simulink model "EMPlanner_cs2018a"  (R2018a)
settings: Solver=ode5  StartTime=0.0  StopTime=30  FixedStep=1/1000  RelTol=1e-3
PreLoadFcn:
  | mbxruntime.callbacks.PreLoadFcn(bdroot);
PostLoadFcn:
  | mbxruntime.callbacks.PostLoadFcn(bdroot);
InitFcn:
  | mbxruntime.callbacks.InitFcn(bdroot);
StartFcn:
  | mbxruntime.callbacks.StartFcn(bdroot);
StopFcn:
  | mbxruntime.callbacks.StopFcn(bdroot);
model workspace (MAT data in the model file):
  mbox_table : struct (value not decoded)
  model_closed = 0
  sim_status = 0
values from neighbouring files (symbols this model uses):
  aubr = [-8 -7.95 -7.9 -7.85 -7.8 -7.75 -7.7 -7.65 -7.6 -7.55 -7.5 -7.45 ... (261 elements, 1x261)]    [table_calibration.mat]
  tablebr = [-1.5 -1.5 -6.69193204056 -6.72439369683 -6.74529114616 -6.75462438856 -6.75239342402 -6.74076432593 -6.71187451024 -6.7106900587 -6.78609036519 -6.73359919607 ... (261261 elements, 1001x261)]    [table_calibration.mat]
  vubr = [0 0.05 0.1 0.15 0.2 0.25 0.3 0.35 0.4 0.45 0.5 0.55 ... (1001 elements, 1x1001)]    [table_calibration.mat]
undefined symbols (not defined in the file or in its folder): c_factor, cf, cr, DiscIntNeverNeededParam, global_path_x, global_path_y, KD_PID_distance, KD_PID_speed, KI_PID_distance, KI_PID_speed, KP_PID_distance, KP_PID_speed, la, lb, LQR_K1, LQR_K2, LQR_K3, LQR_K4, m, rack_displacement, right_wheel_ground, vx_break_point, warningInitialVelocity, x0
libraries: PreScanSimulinkLibrary x39, simulink x19, simulink_extras x11, Solver_SF x1
(part 4 of 11)

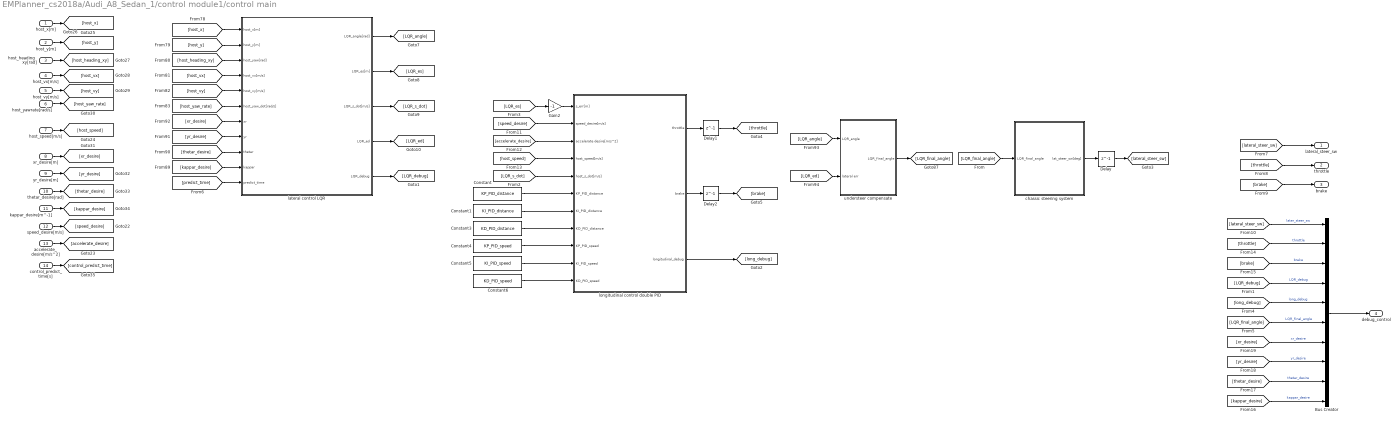
== system EMPlanner_cs2018a/Audi_A8_Sedan_1/control module1/control main ==
  host_x[m] : Inport
  host_y[m] : Inport  Port=2
  host_heading_xy[rad] : Inport  Port=3
  host_vx[m/s] : Inport  Port=4
  host_vy[m/s] : Inport  Port=5
  host_yawrate[rad/s] : Inport  Port=6
  host_speed[m/s] : Inport  Port=7
  xr_desire[m] : Inport  Port=8
  yr_desire[m] : Inport  Port=9
  thetar_desire[rad] : Inport  Port=10
  kappar_desire[m^-1] : Inport  Port=11
  speed_desire[m/s] : Inport  Port=12
  accelerate_desire[m/s^2] : Inport  Port=13
  control_predict_time[s] : Inport  Port=14
  Bus Creator : BusCreator  Inputs=10
  Constant : Constant  Value=KP_PID_distance
  Constant1 : Constant  Value=KI_PID_distance
  Constant3 : Constant  Value=KD_PID_distance
  Constant4 : Constant  Value=KP_PID_speed
  Constant5 : Constant  Value=KI_PID_speed
  Constant6 : Constant  Value=KD_PID_speed
  Delay : Delay  DelayLength=1
  Delay1 : Delay  DelayLength=1
  Delay2 : Delay  DelayLength=1
  Gain2 : Gain  Gain=-1
  chassic steering system : Subsystem
  lateral control LQR : Subsystem
  longitudinal control double PID : Subsystem
  understeer compensate : Subsystem
  lateral_steer_sw : Outport
  throttle : Outport  Port=2
  brake : Outport  Port=3
  debug_control : Outport  Port=4
  wires:
  host_x[m]/1 -> [host_x]
  understeer compensate/1(LQR_final_angle) -> [LQR_final_angle]
  lateral control LQR/1(LQR_angle[rad]) -> [LQR_angle]
  [host_vx] -> lateral control LQR/4(host_vx[m/s])
  thetar_desire[rad]/1 -> [thetar_desire]
  Constant1/1 -> longitudinal control double PID/7(KI_PID_distance)
  [accelerate_desire] -> longitudinal control double PID/3(accelerate desire[m/s^2])
  [host_x] -> lateral control LQR/1(host_x[m])
  [xr_desire] -> lateral control LQR/7(xr)
  accelerate_desire[m/s^2]/1 -> [accelerate_desire]
  [host_y] -> lateral control LQR/2(host_y[m])
  [LQR_s_dot] -> longitudinal control double PID/5(host_s_dot[m/s])
  [yr_desire] -> lateral control LQR/8(yr)
  [LQR_angle] -> understeer compensate/1(LQR_angle)
  xr_desire[m]/1 -> [xr_desire]
  [host_vy] -> lateral control LQR/5(host_vy[m/s])
  lateral control LQR/2(LQR_es[m]) -> [LQR_es]
  host_heading_xy[rad]/1 -> [host_heading_xy]
  [LQR_ed] -> understeer compensate/2(lateral err)
  lateral control LQR/3(LQR_s_dot[m/s]) -> [LQR_s_dot]
  Constant/1 -> longitudinal control double PID/6(KP_PID_distance)
  Constant3/1 -> longitudinal control double PID/8(KD_PID_distance)
  Constant5/1 -> longitudinal control double PID/10(KI_PID_speed)
  Constant4/1 -> longitudinal control double PID/9(KP_PID_speed)
  [host_speed] -> longitudinal control double PID/4(host_speed[m/s])
  [predict_time] -> lateral control LQR/11(predict_time)
  host_vx[m/s]/1 -> [host_vx]
  [speed_desire] -> longitudinal control double PID/2(speed_desire[m/s])
  lateral control LQR/4(LQR_ed) -> [LQR_ed]
  [thetar_desire] -> lateral control LQR/9(thetar)
  [host_heading_xy] -> lateral control LQR/3(host_yaw[rad])
  [kappar_desire] -> lateral control LQR/10(kappar)
  host_yawrate[rad/s]/1 -> [host_yaw_rate]
  kappar_desire[m^-1]/1 -> [kappar_desire]
  yr_desire[m]/1 -> [yr_desire]
  [host_yaw_rate] -> lateral control LQR/6(host_yaw_dot[rad/s])
  host_y[m]/1 -> [host_y]
  host_vy[m/s]/1 -> [host_vy]
  host_speed[m/s]/1 -> [host_speed]
  control_predict_time[s]/1 -> [control_predict_time]
  speed_desire[m/s]/1 -> [speed_desire]
  Constant6/1 -> longitudinal control double PID/11(KD_PID_speed)
  Gain2/1 -> longitudinal control double PID/1(s_err[m])
  [LQR_es] -> Gain2/1
  [LQR_final_angle] -> chassic steering system/1(LQR_final_angle)
  chassic steering system/1(lat_steer_sw[deg]) -> Delay/1
  longitudinal control double PID/1(throttle) -> Delay1/1
  longitudinal control double PID/2(brake) -> Delay2/1
  lateral control LQR/5(LQR_debug) -> [LQR_debug]
  longitudinal control double PID/3(longitudinal_debug) -> [long_debug]
  Delay/1 -> [lateral_steer_sw]
  Delay1/1 -> [throttle]
  Delay2/1 -> [brake]
  [lateral_steer_sw] -> lateral_steer_sw/1
  [throttle] -> throttle/1
  [brake] -> brake/1
  [lateral_steer_sw] -> Bus Creator/1  "later_steer_sw"
  [throttle] -> Bus Creator/2  "throttle"
  [brake] -> Bus Creator/3  "brake"
  [LQR_debug] -> Bus Creator/4  "LQR_debug"
  [long_debug] -> Bus Creator/5  "long_debug"
  [LQR_final_angle] -> Bus Creator/6  "LQR_final_angle"
  Bus Creator/1 -> debug_control/1
  [xr_desire] -> Bus Creator/7  "xr_desire"
  [yr_desire] -> Bus Creator/8  "yr_desire"
  [thetar_desire] -> Bus Creator/9  "thetar_desire"
  [kappar_desire] -> Bus Creator/10  "kappar_desire"

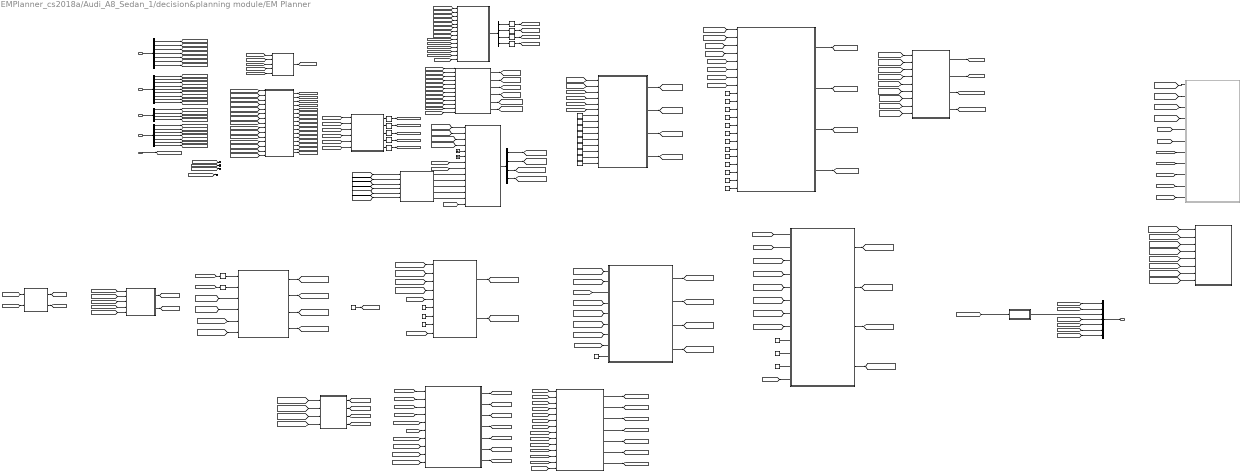
== system EMPlanner_cs2018a/Audi_A8_Sedan_1/decision&planning module/EM Planner ==
  referenceline info : Inport
  location info : Inport  Port=2
  perception info : Inport  Port=3
  pre_planning info : Inport  Port=4
  current time : Inport  Port=5
  Bus Creator : BusCreator  Inputs=7
  Bus Selector : BusSelector  OutputSignals=referenceline_x,referenceline_y,referenceline_heading,referenceline_kappa,origin_match_point_index,origin_x,origin_y
  Bus Selector1 : BusSelector  OutputSignals=host_x,host_y,host_heading_xy,host_vx,host_vy,host_yawrate,host_speed,host_ax,host_ay
  Bus Selector2 : BusSelector  OutputSignals=obs_x_set_gcs,obs_y_set_gcs,obs_velocity_set_gcs,obs_heading_set_gcs
  Bus Selector3 : BusSelector  OutputSignals=trajectory_x_gcs,trajectory_y_gcs,trajectory_heading_gcs,trajectory_kappa_gcs,trajectory_speed_gcs,trajectory_accel_gcs,trajectory_time_gcs
  Bus Selector4 : BusSelector  OutputSignals=s_set,l_set,dl_set,ddl_set
  Bus Selector5 : BusSelector  OutputSignals=s_set,l_set,s_dot_set,l_dot_set
  Cartesian2Frenet : Subsystem
  Cartesian2Frenet1 : Subsystem
  Constant : Constant  Value=1e6
  Constant1 : Constant  Value=2000
  Constant10 : Constant  Value=0.1
  Constant11 : Constant  Value=0.02
  Constant12 : Constant  Value=2
  Constant13 : Constant  Value=25000
  Constant14 : Constant  Value=50
  Constant15 : Constant  Value=20
  Constant{7,16..19,23} (6 alike) : Constant  Value=15
  Constant2 : Constant  Value=2
  Constant20 : Constant  Value=3
  Constant21 : Constant  Value=3
  Constant22 : Constant  Value=1.63
  Constant24 : Constant  Value=4000
  Constant25 : Constant  Value=100
  Constant26 : Constant  Value=10000000
  Constant27 : Constant  Value=0.2*9.8
  Constant28 : Constant  Value=50
  Constant29 : Constant  Value=500
  Constant3 : Constant  Value=3
  Constant4 : Constant  Value=10
  Constant5 : Constant  Value=11
  Constant6 : Constant  Value=4
  Constant8 : Constant
  Constant9 : Constant  Value=10
  Delay : Delay  DelayLength=1
  Delay1 : Delay  DelayLength=1
  Frenet2Cartesian task : MATLAB Function  TreatAsAtomicUnit=on
  Ground : Ground
  Ground1 : Ground
  MATLAB Function : MATLAB Function  TreatAsAtomicUnit=on
  MATLAB Function1 : MATLAB Function  TreatAsAtomicUnit=on
  MATLAB Function2 : MATLAB Function  TreatAsAtomicUnit=on
  MATLAB Function5 : MATLAB Function  TreatAsAtomicUnit=on
  Selector{1..9} (9 alike) : Selector  InputPortWidth=128  IndexOptions=Index vector (dialog)  Indices=1  OutputSizes=1
  Terminator_{1..4} (4 alike) : Terminator
  calc path length and map between point and s : MATLAB Function  TreatAsAtomicUnit=on
  calc plan start info and stitch trajectory : MATLAB Function  TreatAsAtomicUnit=on
  calc speed planning start condition : MATLAB Function  TreatAsAtomicUnit=on
  generate convex space : MATLAB Function  TreatAsAtomicUnit=on
  generate st graph : MATLAB Function  TreatAsAtomicUnit=on
  genrate index to s : MATLAB Function  TreatAsAtomicUnit=on
  increase st point count : MATLAB Function  TreatAsAtomicUnit=on
  obs : Subsystem
  path and speed merge : MATLAB Function  TreatAsAtomicUnit=on
  path decision task : Subsystem
  path planning task : Subsystem
  plot : MATLAB Function  Commented=on  TreatAsAtomicUnit=on
  spee planning with quadratic programming (qp) : MATLAB Function  TreatAsAtomicUnit=on
  speed decision with dynamic planning(dp) : MATLAB Function  TreatAsAtomicUnit=on
  stitch trajectory : MATLAB Function  TreatAsAtomicUnit=on
  EM Planner result : Outport
  wires:
  referenceline info/1 -> Bus Selector/1
  location info/1 -> Bus Selector1/1
  perception info/1 -> Bus Selector2/1
  pre_planning info/1 -> Bus Selector3/1
  current time/1 -> [current_time]
  Bus Selector3/1 -> [pre_trajectory_x_gcs]  "<trajectory_x_gcs>"
  Bus Selector3/2 -> [pre_trajectory_y_gcs]  "<trajectory_y_gcs>"
  Bus Selector3/3 -> [pre_trajectory_heading_gcs]  "<trajectory_heading_gcs>"
  Bus Selector3/4 -> [pre_trajectory_kappa_gcs]  "<trajectory_kappa_gcs>"
  Bus Selector3/5 -> [pre_trajectory_speed_gcs]  "<trajectory_speed_gcs>"
  Bus Selector3/6 -> [pre_trajectory_accel_gcs]  "<trajectory_accel_gcs>"
  Bus Selector3/7 -> [pre_trajectory_time]  "<trajectory_time_gcs>"
  Bus Selector2/1 -> [obs_x_set_gcs]  "<obs_x_set_gcs>"
  Bus Selector2/2 -> [obs_y_set_gcs]  "<obs_y_set_gcs>"
  Bus Selector2/3 -> [obs_velocity_set_gcs]  "<obs_velocity_set_gcs>"
  Bus Selector2/4 -> [obs_heading_set_gcs]  "<obs_heading_set_gcs>"
  Bus Selector1/1 -> [host_x]  "<host_x>"
  Bus Selector1/2 -> [host_y]  "<host_y>"
  Bus Selector1/3 -> [host_heading_xy]  "<host_heading_xy>"
  Bus Selector1/4 -> [host_vx_vcs]  "<host_vx>"
  Bus Selector1/5 -> [host_vy_vcs]  "<host_vy>"
  Bus Selector1/6 -> [host_yawrate]  "<host_yawrate>"
  Bus Selector1/7 -> [host_speed]  "<host_speed>"
  Bus Selector1/8 -> [host_ax_vcs]  "<host_ax>"
  Bus Selector1/9 -> [host_ay_vcs]  "<host_ay>"
  Bus Selector/1 -> [referenceline_x]  "<referenceline_x>"
  Bus Selector/2 -> [referenceline_y]  "<referenceline_y>"
  Bus Selector/3 -> [referenceline_heading]  "<referenceline_heading>"
  Bus Selector/4 -> [referenceline_kappa]  "<referenceline_kappa>"
  [host_ay_vcs] -> calc plan start info and stitch trajectory/15(host_ay)
  [host_ax_vcs] -> calc plan start info and stitch trajectory/14(host_ax)
  [host_vy_vcs] -> calc plan start info and stitch trajectory/13(host_vy)
  [host_vx_vcs] -> calc plan start info and stitch trajectory/12(host_vx)
  [host_heading_xy] -> calc plan start info and stitch trajectory/11(host_heading_xy)
  [host_y] -> calc plan start info and stitch trajectory/10(host_y)
  [host_x] -> calc plan start info and stitch trajectory/9(host_x)
  [current_time] -> calc plan start info and stitch trajectory/8(current_time)
  [pre_trajectory_x_gcs] -> calc plan start info and stitch trajectory/1(pre_trajectory_x)
  [pre_trajectory_y_gcs] -> calc plan start info and stitch trajectory/2(pre_trajectory_y)
  [pre_trajectory_time] -> calc plan start info and stitch trajectory/7(pre_trajectory_time)
  [pre_trajectory_accel_gcs] -> calc plan start info and stitch trajectory/6(pre_trajectory_accel)
  [pre_trajectory_speed_gcs] -> calc plan start info and stitch trajectory/5(pre_trajectory_velocity)
  [pre_trajectory_kappa_gcs] -> calc plan start info and stitch trajectory/4(pre_trajectory_kappa)
  [pre_trajectory_heading_gcs] -> calc plan start info and stitch trajectory/3(pre_trajectory_heading)
  calc plan start info and stitch trajectory/1(plan_start_x) -> [plan_start_x_gcs]
  calc plan start info and stitch trajectory/2(plan_start_y) -> [plan_start_y_gcs]
  calc plan start info and stitch trajectory/3(plan_start_heading) -> [plan_start_heading_gcs]
  calc plan start info and stitch trajectory/4(plan_start_kappa) -> [plan_start_kappa_gcs]
  calc plan start info and stitch trajectory/5(plan_start_vx) -> [plan_start_vx_gcs]
  calc plan start info and stitch trajectory/6(plan_start_vy) -> [plan_start_vy_gcs]
  calc plan start info and stitch trajectory/7(plan_start_ax) -> [plan_start_ax_gcs]
  calc plan start info and stitch trajectory/8(plan_start_ay) -> [plan_start_ay_gcs]
  calc plan start info and stitch trajectory/9(plan_start_time) -> [plan_start_time]
  calc plan start info and stitch trajectory/10(stitch_x) -> [stitch_x_gcs]
  calc plan start info and stitch trajectory/11(stitch_y) -> [stitch_y_gcs]
  calc plan start info and stitch trajectory/12(stitch_heading) -> [stitch_heading_gcs]
  calc plan start info and stitch trajectory/13(stitch_kappa) -> [stitch_kappa_gcs]
  calc plan start info and stitch trajectory/14(stitch_speed) -> [stitch_speed_gcs]
  calc plan start info and stitch trajectory/15(stitch_accel) -> [stitch_accel_gcs]
  calc plan start info and stitch trajectory/16(stitch_time) -> [stitch_time]
  Bus Selector/5 -> [origin_match_point_index]  "<origin_match_point_index>"
  Bus Selector/6 -> [origin_x]  "<origin_x>"
  Bus Selector/7 -> [origin_y]  "<origin_y>"
  [referenceline_x] -> genrate index to s/1(path_x)
  [referenceline_y] -> genrate index to s/2(path_y)
  [origin_x] -> genrate index to s/3(origin_x)
  [origin_y] -> genrate index to s/4(origin_y)
  [origin_match_point_index] -> genrate index to s/5(origin_match_point_index)
  genrate index to s/1(index2s) -> [index2s]
  MATLAB Function2/5(proj_kappa_set) -> Selector5/1
  MATLAB Function2/3(proj_y_set) -> Selector3/1
  MATLAB Function2/1(match_point_index_set) -> Selector1/1
  MATLAB Function2/4(proj_heading_set) -> Selector4/1
  MATLAB Function2/2(proj_x_set) -> Selector2/1
  [plan_start_x_gcs] -> MATLAB Function2/1(x_set)
  [plan_start_y_gcs] -> MATLAB Function2/2(y_set)
  [referenceline_x] -> MATLAB Function2/3(frenet_path_x)
  [referenceline_y] -> MATLAB Function2/4(frenet_path_y)
  [referenceline_heading] -> MATLAB Function2/5(frenet_path_heading)
  [referenceline_kappa] -> MATLAB Function2/6(frenet_path_kappa)
  Selector1/1 -> [plan_start_match_point_index]
  Selector2/1 -> [plan_start_proj_x]
  Selector3/1 -> [plan_start_proj_y]
  Selector4/1 -> [plan_start_proj_heading]
  Selector5/1 -> [plan_start_proj_kappa]
  [plan_start_y_gcs] -> Cartesian2Frenet/2(y_set)
  [plan_start_x_gcs] -> Cartesian2Frenet/1(x_set)
  [plan_start_vx_gcs] -> Cartesian2Frenet/3(vx_set)
  [plan_start_vy_gcs] -> Cartesian2Frenet/4(vy_set)
  [plan_start_ax_gcs] -> Cartesian2Frenet/5(ax_set)
  [plan_start_ay_gcs] -> Cartesian2Frenet/6(ay_set)
  [referenceline_x] -> Cartesian2Frenet/7(frenet_path_x)
  [referenceline_y] -> Cartesian2Frenet/8(frenet_path_y)
  [plan_start_match_point_index] -> Cartesian2Frenet/9(proj_match_point_index_set)
  [plan_start_proj_x] -> Cartesian2Frenet/10(proj_x_set)
  [plan_start_proj_y] -> Cartesian2Frenet/11(proj_y_set)
  [plan_start_proj_heading] -> Cartesian2Frenet/12(proj_heading_set)
  [plan_start_proj_kappa] -> Cartesian2Frenet/13(proj_kappa_set)
  Cartesian2Frenet/1(Cartesian2FrenetOut) -> Bus Selector4/1
  Bus Selector4/4 -> Selector9/1  "<ddl_set>"
  Bus Selector4/3 -> Selector8/1  "<dl_set>"
  Bus Selector4/2 -> Selector7/1  "<l_set>"
  Bus Selector4/1 -> Selector6/1  "<s_set>"
  Selector6/1 -> [plan_start_s]
  Selector7/1 -> [plan_start_l]
  Selector8/1 -> [plan_start_dl]
  Selector9/1 -> [plan_start_ddl]
  [index2s] -> Cartesian2Frenet/14(index2s)
  [host_x] -> obs/1(host_x)
  [host_y] -> obs/2(host_y)
  [host_heading_xy] -> obs/3(host_heading_xy)
  [obs_x_set_gcs] -> obs/4(obs_x_set_gcs)
  [obs_y_set_gcs] -> obs/5(obs_y_set_gcs)
  [obs_velocity_set_gcs] -> obs/6(obs_velocity_set_gcs)
  [obs_heading_set_gcs] -> obs/7(obs_heading_set_gcs)
  [referenceline_x] -> obs/8(referenceline_x)
  [referenceline_y] -> obs/9(referenceline_y)
  [referenceline_heading] -> obs/10(referenceline_heading)
  [referenceline_kappa] -> obs/11(referenceline_kappa)
  [index2s] -> obs/12(index2s)
  obs/1(static_obs_s_set) -> [static_obs_s_set]
  obs/2(static_obs_l_set) -> [static_obs_l_set]
  path and speed merge/7(trajectory_time) -> [trajectory_time]
  path and speed merge/1(trajectory_x) -> [trajectory_x]
  [trajectory_speed] -> stitch trajectory/5(trajectory_speed)
  path and speed merge/4(trajectory_kappa) -> [trajectory_kappa]
  [plan_start_vy_gcs] -> calc speed planning start condition/2(plan_start_vy)
  [stitch_time] -> stitch trajectory/14(stitch_time)
  calc path length and map between point and s/2(path_index2s) -> [path_index2s]
  [plan_start_heading_gcs] -> calc speed planning start condition/5(plan_start_heading)
  Bus Creator/1 -> EM Planner result/1
  [trajectory_x_final] -> Bus Creator/1  "trajectory_x_gcs"
  stitch trajectory/4(trajectory_kappa_final) -> [trajectory_kappa_final]
  [plan_start_ax_gcs] -> calc speed planning start condition/3(plan_start_ax)
  calc speed planning start condition/1(plan_start_s_dot) -> [plan_start_s_dot]
  [plan_start_ay_gcs] -> calc speed planning start condition/4(plan_start_ay)
  [stitch_speed_gcs] -> stitch trajectory/12(stitch_speed)
  [trajectory_time_final] -> Bus Creator/7  "trajectory_time_gcs"
  [stitch_x_gcs] -> stitch trajectory/8(stitch_x)
  stitch trajectory/1(trajectory_x_final) -> [trajectory_x_final]
  [trajectory_accel_final] -> Bus Creator/6  "trajectory_accel_gcs"
  [stitch_heading_gcs] -> stitch trajectory/10(stitch_heading)
  [trajectory_speed_final] -> Bus Creator/5  "trajectory_speed_gcs"
  [stitch_y_gcs] -> stitch trajectory/9(stitch_y)
  stitch trajectory/6(trajectory_accel_final) -> [trajectory_accel_final]
  [plan_start_vx_gcs] -> calc speed planning start condition/1(plan_start_vx)
  [trajectory_heading_final] -> MATLAB Function/1(trajectory_heading_final)
  [trajectory_accel] -> stitch trajectory/6(trajectory_accel)
  [trajectory_kappa] -> stitch trajectory/4(trajectory_kappa)
  [trajectory_x_init] -> path and speed merge/7(trajectory_x_init)
  stitch trajectory/2(trajectory_y_final) -> [trajectory_y_final]
  stitch trajectory/3(trajectory_heading_final) -> [trajectory_heading_final]
  [trajectory_kappa_final] -> Bus Creator/4  "trajectory_kappa_gcs"
  path and speed merge/3(trajectory_heading) -> [trajectory_heading]
  stitch trajectory/5(trajectory_speed_final) -> [trajectory_speed_final]
  [trajectory_y_final] -> Bus Creator/2  "trajectory_y_gcs"
  [trajectory_y] -> stitch trajectory/2(trajectory_y)
  calc path length and map between point and s/1(path_s_end) -> [path_s_end]
  calc speed planning start condition/2(plan_start_s_dot2) -> [plan_start_s_dot2]
  [trajectory_kappa_init] -> path and speed merge/10(trajectory_kappa_init)
  [stitch_accel_gcs] -> stitch trajectory/13(stitch_accel)
  [trajectory_x] -> stitch trajectory/1(trajectory_x)
  [trajectory_y_init] -> calc path length and map between point and s/2(trajectory_y)
  path and speed merge/6(trajectory_accel) -> [trajectory_accel]
  [stitch_kappa_gcs] -> stitch trajectory/11(stitch_kappa)
  [path_index2s] -> path and speed merge/6(path_s)
  path and speed merge/2(trajectory_y) -> [trajectory_y]
  [trajectory_heading_init] -> path and speed merge/9(trajectory_heading_init)
  [plan_start_time] -> path and speed merge/5(current_time)
  path and speed merge/5(trajectory_speed) -> [trajectory_speed]
  [trajectory_y_init] -> path and speed merge/8(trajectory_y_init)
  [trajectory_time] -> stitch trajectory/7(trajectory_time)
  [trajectory_heading] -> stitch trajectory/3(trajectory_heading)
  [trajectory_x_init] -> calc path length and map between point and s/1(trajectory_x)
  [index2s] -> Frenet2Cartesian task/9(index2s)
  [referenceline_x] -> Frenet2Cartesian task/5(frenet_path_x)
  [referenceline_y] -> Frenet2Cartesian task/6(frenet_path_y)
  [referenceline_heading] -> Frenet2Cartesian task/7(frenet_path_heading)
  [referenceline_kappa] -> Frenet2Cartesian task/8(frenet_path_kappa)
  Frenet2Cartesian task/1(x_set) -> [trajectory_x_init]
  Frenet2Cartesian task/2(y_set) -> [trajectory_y_init]
  Frenet2Cartesian task/3(heading_set) -> [trajectory_heading_init]
  Frenet2Cartesian task/4(kappa_set) -> [trajectory_kappa_init]
  [dp_path_s_final] -> plot/1(dp_s)
  [dp_path_l_final] -> plot/2(dp_l)
  [l_min] -> plot/5(l_min)
  [l_max] -> plot/6(l_max)
  [plan_start_dl] -> plot/11(start_dl)
  [plan_start_l] -> plot/10(start_l)
  [plan_start_s] -> plot/9(start_s)
  [static_obs_s_set] -> plot/7(obs_s_set)
  [static_obs_l_set] -> plot/8(obs_l_set)
  path decision task/1(dp_path_s_final) -> [dp_path_s_final]
  path decision task/2(dp_path_l_final) -> [dp_path_l_final]
  path decision task/3(dp_path_dl_final) -> [dp_path_dl_final]
  path decision task/4(dp_path_ddl_final) -> [dp_path_ddl_final]
  [static_obs_s_set] -> path decision task/1(static_obs_s_set)
  [static_obs_l_set] -> path decision task/2(static_obs_l_set)
  [plan_start_ddl] -> path decision task/6(plan_start_ddl)
  [plan_start_dl] -> path decision task/5(plan_start_dl)
  [plan_start_l] -> path decision task/4(plan_start_l)
  [plan_start_s] -> path decision task/3(plan_start_s)
  [dp_path_s_final] -> path planning task/1(dp_path_s_final)
  [dp_path_l_final] -> path planning task/2(dp_path_l_final)
  [plan_start_l] -> path planning task/6(plan_start_l)
  [plan_start_ddl] -> path planning task/8(plan_start_ddl)
  [plan_start_dl] -> path planning task/7(plan_start_dl)
  Constant22/1 -> path planning task/19(host_w)
  Constant21/1 -> path planning task/18(host_d2)
  Constant20/1 -> path planning task/17(host_d1)
  Constant19/1 -> path planning task/16(qp_cost_end_ddl)
  Constant18/1 -> path planning task/15(qp_cost_end_dl)
  Constant17/1 -> path planning task/14(qp_cost_endl)
  Constant16/1 -> path planning task/13(qp_cost_centre)
  Constant15/1 -> path planning task/12(qp_cost_dddl)
  Constant14/1 -> path planning task/11(qp_cost_ddl)
  Constant13/1 -> path planning task/10(qp_cost_dl)
  Constant12/1 -> path planning task/9(qp_cost_l)
  Constant8/1 -> path decision task/15(dp_sample_l)
  Constant7/1 -> path decision task/14(dp_sample_s)
  Constant6/1 -> path decision task/13(dp_col)
  Constant5/1 -> path decision task/12(dp_row)
  Constant4/1 -> path decision task/11(dp_cost_ref)
  Constant3/1 -> path decision task/10(dp_cost_dddl)
  Constant/1 -> path decision task/7(dp_cost_collision)
  Constant1/1 -> path decision task/8(dp_cost_dl)
  Constant2/1 -> path decision task/9(dp_cost_ddl)
  [static_obs_s_set] -> path planning task/3(static_obs_s_set)
  [static_obs_l_set] -> path planning task/4(static_obs_l_set)
  Constant10/1 -> path planning task/20(delta_dl_max)
  Constant11/1 -> path planning task/21(delta_ddl_max)
  path planning task/1(qp_path_s_final) -> [qp_path_s_final]
  path planning task/2(qp_path_l_final) -> [qp_path_l_final]
  path planning task/3(qp_path_dl_final) -> [qp_path_dl_final]
  path planning task/4(qp_path_ddl_final) -> [qp_path_ddl_final]
  [qp_path_ddl_final] -> Frenet2Cartesian task/4(ddl_set)
  [qp_path_l_final] -> Frenet2Cartesian task/2(l_set)
  [qp_path_dl_final] -> Frenet2Cartesian task/3(dl_set)
  [qp_path_s_final] -> Frenet2Cartesian task/1(s_set)
  [qp_path_s_final] -> plot/3(qp_s)
  [qp_path_l_final] -> plot/4(qp_l)
  [plan_start_s] -> path planning task/5(plan_start_s)
  MATLAB Function/1(y) -> Bus Creator/3  "trajectory_heading_gcs"
  obs/3(dynamic_obs_x_set) -> [dynamic_obs_x_set]
  obs/4(dynamic_obs_y_set) -> [dynamic_obs_y_set]
  obs/5(dynamic_obs_vx_set) -> [dynamic_obs_vx_set]
  obs/6(dynamic_obs_vy_set) -> [dynamic_obs_vy_set]
  increase st point count/3(s_dot2) -> [s_dot2]
  increase st point count/2(s_dot) -> [s_dot]
  increase st point count/1(s) -> [s]
  increase st point count/4(relative_time) -> [relative_time]
  [s_dot] -> path and speed merge/2(s_dot)
  [s] -> path and speed merge/1(s)
  [s_dot2] -> path and speed merge/3(s_dot2)
  [relative_time] -> path and speed merge/4(relative_time)
  [dynamic_obs_vy_set] -> Cartesian2Frenet1/4(vy_set)
  [dynamic_obs_vx_set] -> Cartesian2Frenet1/3(vx_set)
  [dynamic_obs_y_set] -> Cartesian2Frenet1/2(y_set)
  [dynamic_obs_x_set] -> Cartesian2Frenet1/1(x_set)
  Ground/1 -> Cartesian2Frenet1/5(ax_set)
  Ground1/1 -> Cartesian2Frenet1/6(ay_set)
  [trajectory_x_init] -> Cartesian2Frenet1/7(frenet_path_x)
  [trajectory_y_init] -> Cartesian2Frenet1/8(frenet_path_y)
  MATLAB Function1/1(match_point_index_set) -> Cartesian2Frenet1/9(proj_match_point_index_set)
  MATLAB Function1/2(proj_x_set) -> Cartesian2Frenet1/10(proj_x_set)
  MATLAB Function1/3(proj_y_set) -> Cartesian2Frenet1/11(proj_y_set)
  MATLAB Function1/4(proj_heading_set) -> Cartesian2Frenet1/12(proj_heading_set)
  MATLAB Function1/5(proj_kappa_set) -> Cartesian2Frenet1/13(proj_kappa_set)
  [trajectory_x_init] -> MATLAB Function1/3(frenet_path_x)
  [trajectory_y_init] -> MATLAB Function1/4(frenet_path_y)
  [trajectory_heading_init] -> MATLAB Function1/5(frenet_path_heading)
  [trajectory_kappa_init] -> MATLAB Function1/6(frenet_path_kappa)
  [dynamic_obs_y_set] -> MATLAB Function1/2(y_set)
  [dynamic_obs_x_set] -> MATLAB Function1/1(x_set)
  Cartesian2Frenet1/1(Cartesian2FrenetOut) -> Bus Selector5/1
  Bus Selector5/1 -> [dynamic_obs_s_set]  "<s_set>"
  Bus Selector5/2 -> [dynamic_obs_l_set]  "<l_set>"
  Bus Selector5/3 -> [dynamic_obs_s_dot_set]  "<s_dot_set>"
  Bus Selector5/4 -> [dynamic_obs_l_dot_set]  "<l_dot_set>"
  [path_index2s] -> Cartesian2Frenet1/14(index2s)
  [s] -> Delay/1
  [relative_time] -> Delay1/1
  Delay/1 -> generate st graph/1(pre_trajectory_s)
  Delay1/1 -> generate st graph/2(pre_trajectory_t)
  stitch trajectory/7(trajectory_time_final) -> [trajectory_time_final]
  [dynamic_obs_s_set] -> generate st graph/3(dynamic_obs_s_set)
  [dynamic_obs_l_set] -> generate st graph/4(dynamic_obs_l_set)
  [dynamic_obs_s_dot_set] -> generate st graph/5(dynamic_obs_s_dot_set)
  [dynamic_obs_l_dot_set] -> generate st graph/6(dynamic_obs_l_dot_set)
  generate st graph/1(obs_st_s_in_set) -> [obs_st_s_in_set]
  generate st graph/3(obs_st_t_in_set) -> [obs_st_t_in_set]
  generate st graph/4(obs_st_t_out_set) -> [obs_st_t_out_set]
  generate st graph/2(obs_st_s_out_set) -> [obs_st_s_out_set]
  [obs_st_s_in_set] -> speed decision with dynamic planning(dp)/1(obs_st_s_in_set)
  [obs_st_s_out_set] -> speed decision with dynamic planning(dp)/2(obs_st_s_out_set)
  [obs_st_t_in_set] -> speed decision with dynamic planning(dp)/3(obs_st_t_in_set)
  [obs_st_t_out_set] -> speed decision with dynamic planning(dp)/4(obs_st_t_out_set)
  Constant24/1 -> speed decision with dynamic planning(dp)/6(w_cost_ref_speed)
  Constant25/1 -> speed decision with dynamic planning(dp)/7(w_cost_accel)
  Constant26/1 -> speed decision with dynamic planning(dp)/8(w_cost_obs)
  [plan_start_s_dot] -> speed decision with dynamic planning(dp)/9(plan_start_s_dot)
  [path_index2s] -> generate convex space/3(path_index2s)
  speed decision with dynamic planning(dp)/2(dp_speed_t) -> [dp_speed_t]
  [dp_speed_s] -> generate convex space/1(dp_speed_s)
  [dp_speed_t] -> generate convex space/2(dp_speed_t)
  [obs_st_s_in_set] -> generate convex space/4(obs_st_s_in_set)
  [obs_st_t_out_set] -> generate convex space/7(obs_st_t_out_set)
  [obs_st_t_in_set] -> generate convex space/6(obs_st_t_in_set)
  [obs_st_s_out_set] -> generate convex space/5(obs_st_s_out_set)
  [trajectory_kappa_init] -> generate convex space/8(trajectory_kappa_init)
  Constant27/1 -> generate convex space/9(max_lateral_accel)
  generate convex space/1(s_lb) -> [s_lb]
  generate convex space/2(s_ub) -> [s_ub]
  generate convex space/3(s_dot_lb) -> [s_dot_lb]
  generate convex space/4(s_dot_ub) -> [s_dot_ub]
  speed decision with dynamic planning(dp)/1(dp_speed_s) -> [dp_speed_s]
  [obs_st_s_in_set] -> MATLAB Function5/5(obs_s_in_set)
  [obs_st_s_out_set] -> MATLAB Function5/6(obs_s_out_set)
  [obs_st_t_in_set] -> MATLAB Function5/7(obs_t_in_set)
  [obs_st_t_out_set] -> MATLAB Function5/8(obs_t_out_set)
  [plan_start_s_dot] -> spee planning with quadratic programming (qp)/1(plan_start_s_dot)
  [dp_speed_s] -> spee planning with quadratic programming (qp)/3(dp_speed_s)
  [dp_speed_t] -> spee planning with quadratic programming (qp)/4(dp_speed_t)
  [s_lb] -> spee planning with quadratic programming (qp)/5(s_lb)
  [s_ub] -> spee planning with quadratic programming (qp)/6(s_ub)
  [s_dot_lb] -> spee planning with quadratic programming (qp)/7(s_dot_lb)
  [s_dot_ub] -> spee planning with quadratic programming (qp)/8(s_dot_ub)
  spee planning with quadratic programming (qp)/1(qp_s_init) -> [qp_s_init]
  spee planning with quadratic programming (qp)/2(qp_s_dot_init) -> [qp_s_dot_init]
  spee planning with quadratic programming (qp)/3(qp_s_dot2_init) -> [qp_s_dot2_init]
  spee planning with quadratic programming (qp)/4(relative_time_init) -> [relative_time_init]
  [qp_s_init] -> increase st point count/1(s_init)
  [qp_s_dot2_init] -> increase st point count/3(s_dot2_init)
  [qp_s_dot_init] -> increase st point count/2(s_dot_init)
  [relative_time_init] -> increase st point count/4(relative_time_init)
  Constant9/1 -> spee planning with quadratic programming (qp)/9(w_cost_s_dot2)
  Constant28/1 -> spee planning with quadratic programming (qp)/10(w_cost_v_ref)
  Constant29/1 -> spee planning with quadratic programming (qp)/11(w_cost_jerk)
  [plan_start_s_dot2] -> spee planning with quadratic programming (qp)/2(plan_start_s_dot2)
  [dp_speed_t] -> MATLAB Function5/2(dp_speed_t)
  [dp_speed_s] -> MATLAB Function5/1(dp_speed_s)
  [qp_s_init] -> MATLAB Function5/3(qp_speed_s)
  [relative_time_init] -> MATLAB Function5/4(qp_speed_t)
  Constant23/1 -> [reference_speed]
  [reference_speed] -> speed decision with dynamic planning(dp)/5(reference_speed_unlimit)
  [reference_speed] -> spee planning with quadratic programming (qp)/12(speed_reference)
  [pre_trajectory_x_gcs] -> Terminator_1/1
  [pre_trajectory_y_gcs] -> Terminator_2/1
  [pre_trajectory_speed_gcs] -> Terminator_3/1
  [pre_trajectory_time] -> Terminator_4/1

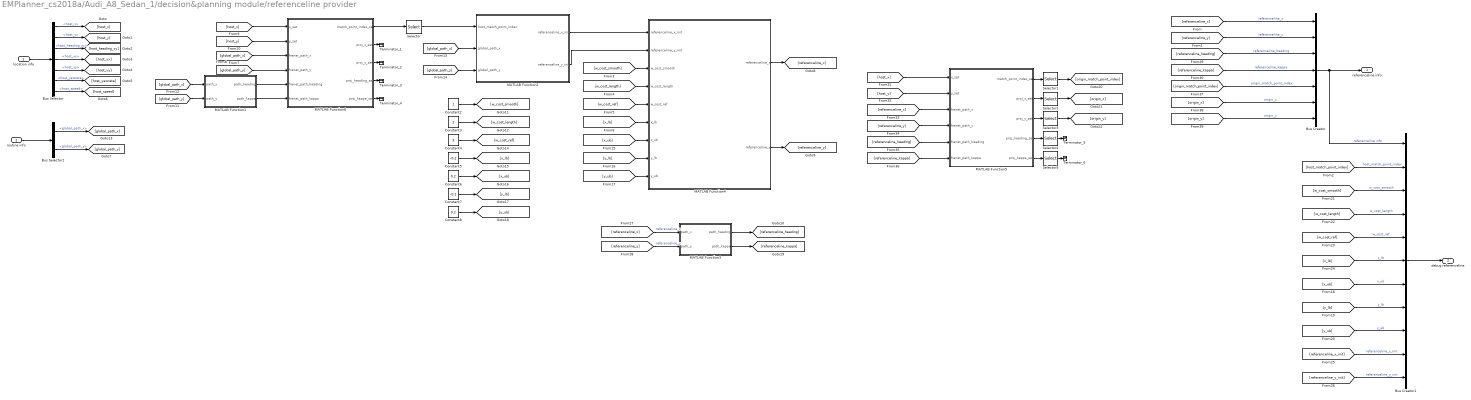
== system EMPlanner_cs2018a/Audi_A8_Sedan_1/decision&planning module/referenceline provider ==
  location info : Inport
  routine info : Inport  Port=2
  Bus Creator : BusCreator  Inputs=7
  Bus Creator1 : BusCreator  Inputs=11
  Bus Selector : BusSelector  OutputSignals=host_x,host_y,host_heading_xy,host_vx,host_vy,host_yawrate,host_speed
  Bus Selector1 : BusSelector  OutputSignals=global_path_x,global_path_y
  Constant2 : Constant
  Constant3 : Constant  Value=2
  Constant4 : Constant  Value=3
  Constant5 : Constant  Value=-0.2
  Constant6 : Constant  Value=0.2
  Constant7 : Constant  Value=-0.2
  Constant8 : Constant  Value=0.2
  MATLAB Function1 : MATLAB Function  TreatAsAtomicUnit=on
  MATLAB Function2 : MATLAB Function  TreatAsAtomicUnit=on
  MATLAB Function3 : MATLAB Function  TreatAsAtomicUnit=on
  MATLAB Function4 : MATLAB Function  TreatAsAtomicUnit=on
  MATLAB Function5 : MATLAB Function  TreatAsAtomicUnit=on
  MATLAB Function6 : MATLAB Function  TreatAsAtomicUnit=on
  Selector{,1..5} (6 alike) : Selector  InputPortWidth=128  IndexOptions=Index vector (dialog)  Indices=1  OutputSizes=1
  Terminator_{1..6} (6 alike) : Terminator
  referenceline info : Outport
  debug referenceline : Outport  Port=2
  wires:
  [global_path_x] -> MATLAB Function2/2(global_path_x)
  [host_x] -> MATLAB Function6/1(x_set)
  MATLAB Function1/2(path_kappa) -> MATLAB Function6/6(frenet_path_kappa)
  MATLAB Function1/1(path_heading) -> MATLAB Function6/5(frenet_path_heading)
  [global_path_y] -> MATLAB Function6/4(frenet_path_y)
  [global_path_x] -> MATLAB Function6/3(frenet_path_x)
  [host_y] -> MATLAB Function6/2(y_set)
  [global_path_y] -> MATLAB Function1/2(path_y)
  [global_path_x] -> MATLAB Function1/1(path_x)
  Selector/1 -> MATLAB Function2/1(host_match_point_index)
  MATLAB Function6/1(match_point_index_set) -> Selector/1
  [global_path_y] -> MATLAB Function2/3(global_path_y)
  MATLAB Function2/1(referenceline_x_init) -> MATLAB Function4/1(referenceline_x_init)
  Bus Selector/5 -> [host_vy]  "<host_vy>"
  Bus Selector/1 -> [host_x]  "<host_x>"
  Bus Selector/2 -> [host_y]  "<host_y>"
  Bus Selector/3 -> [host_heading_xy]  "<host_heading_xy>"
  Bus Selector/4 -> [host_vx]  "<host_vx>"
  Bus Selector/7 -> [host_speed]  "<host_speed>"
  Bus Selector/6 -> [host_yawrate]  "<host_yawrate>"
  location info/1 -> Bus Selector/1
  Bus Selector1/2 -> [global_path_y]  "<global_path_y>"
  Bus Selector1/1 -> [global_path_x]  "<global_path_x>"
  routine info/1 -> Bus Selector1/1
  MATLAB Function4/1(referenceline_x) -> [referenceline_x]
  MATLAB Function4/2(referenceline_y) -> [referenceline_y]
  [referenceline_x] -> Bus Creator/1  "referenceline_x"
  [referenceline_y] -> Bus Creator/2  "referenceline_y"
  Bus Creator1/1 -> debug referenceline/1
  Bus Creator/1 -> Bus Creator1/1, referenceline info/1  "referenceline info"
  Constant2/1 -> [w_cost_smooth]
  Constant3/1 -> [w_cost_length]
  Constant8/1 -> [y_ub]
  Constant7/1 -> [y_lb]
  Constant6/1 -> [x_ub]
  Constant5/1 -> [x_lb]
  Constant4/1 -> [w_cost_ref]
  [w_cost_smooth] -> MATLAB Function4/3(w_cost_smooth)
  [w_cost_length] -> MATLAB Function4/4(w_cost_length)
  [w_cost_ref] -> MATLAB Function4/5(w_cost_ref)
  [x_lb] -> MATLAB Function4/6(x_lb)
  [x_ub] -> MATLAB Function4/7(x_ub)
  [y_lb] -> MATLAB Function4/8(y_lb)
  [y_ub] -> MATLAB Function4/9(y_ub)
  MATLAB Function2/2(referenceline_y_init) -> MATLAB Function4/2(referenceline_y_init)
  [w_cost_ref] -> Bus Creator1/5  "w_cost_ref"
  [x_lb] -> Bus Creator1/6  "x_lb"
  [w_cost_length] -> Bus Creator1/4  "w_cost_length"
  [x_ub] -> Bus Creator1/7  "x_ub"
  [w_cost_smooth] -> Bus Creator1/3  "w_cost_smooth"
  [y_lb] -> Bus Creator1/8  "y_lb"
  [host_match_point_index] -> Bus Creator1/2  "host_match_point_index"
  [y_ub] -> Bus Creator1/9  "y_ub"
  [referenceline_x_init] -> Bus Creator1/10  "referenceline_x_init"
  [referenceline_y_init] -> Bus Creator1/11  "referenceline_y_init"
  [referenceline_x] -> MATLAB Function3/1(path_x)  "referenceline_x"
  [referenceline_y] -> MATLAB Function3/2(path_y)  "referenceline_y"
  MATLAB Function3/1(path_heading) -> [referenceline_heading]
  MATLAB Function3/2(path_kappa) -> [referenceline_kappa]
  [referenceline_kappa] -> Bus Creator/4  "referenceline_kappa"
  [referenceline_heading] -> Bus Creator/3  "referenceline_heading"
  [host_x] -> MATLAB Function5/1(x_set)
  [host_y] -> MATLAB Function5/2(y_set)
  [referenceline_x] -> MATLAB Function5/3(frenet_path_x)
  [referenceline_y] -> MATLAB Function5/4(frenet_path_y)
  [referenceline_heading] -> MATLAB Function5/5(frenet_path_heading)
  [referenceline_kappa] -> MATLAB Function5/6(frenet_path_kappa)
  MATLAB Function5/1(match_point_index_set) -> Selector1/1
  MATLAB Function5/2(proj_x_set) -> Selector2/1
  MATLAB Function5/3(proj_y_set) -> Selector3/1
  MATLAB Function5/4(proj_heading_set) -> Selector4/1
  MATLAB Function5/5(proj_kappa_set) -> Selector5/1
  Selector1/1 -> [origin_match_point_index]
  Selector2/1 -> [origin_x]
  Selector3/1 -> [origin_y]
  [origin_match_point_index] -> Bus Creator/5  "origin_match_point_index"
  [origin_x] -> Bus Creator/6  "origin_x"
  [origin_y] -> Bus Creator/7  "origin_y"
  MATLAB Function6/2(proj_x_set) -> Terminator_1/1
  MATLAB Function6/3(proj_y_set) -> Terminator_2/1
  MATLAB Function6/4(proj_heading_set) -> Terminator_3/1
  MATLAB Function6/5(proj_kappa_set) -> Terminator_4/1
  Selector4/1 -> Terminator_5/1
  Selector5/1 -> Terminator_6/1

== system EMPlanner_cs2018a/Audi_A8_Sedan_2/Dynamics_Simple/Chassis ==
  TransmissionTorque_[Nm] : Inport
  BrakePressure_[bar] : Inport  Port=2
  DeltaSteer_[deg] : Inport  Port=3
  Initial_Vx_[m s-1] : Inport  Port=4
  Abs : Abs
  Bicycle_model_[XYZ] : Subsystem
      mask Display: image(imread('Bicycle_model.png'));
  Constant3 : Constant  Value=[0 0]
  Constant4 : Constant  Value=[0 0]
  Degrees to Radians : simulink_extras/Transformations/Degrees to Radians
  FinalDriveRatio : Gain  Gain=p.Rfd  SaturateOnIntegerOverflow=on  OutDataTypeStr=Inherit: Same as input  ParamDataTypeStr=Inherit: Same as input
  "FinalDriveRatio " : Gain  Gain=p.Rfd  SaturateOnIntegerOverflow=on  OutDataTypeStr=Inherit: Same as input  ParamDataTypeStr=Inherit: Same as input
  FrontTyre : Subsystem
      mask Display: image(imread('Tyre.png'));
  Gain : Gain  Gain=2*pi/60
  MuxDynState : Subsystem
  Power Assisted Steering : Subsystem
  Product : Product  RndMeth=Zero
  RearTyre : Subsystem
      mask Display: image(imread('Tyre.png'));
  SteerRatio : Gain  Gain=1/p.SteerRatio
  Terminator4 : Terminator
  "[ms-1 --> rpm]" : Gain  Gain=60/(2*pi*p.Rw)  SaturateOnIntegerOverflow=on  OutDataTypeStr=Inherit: Same as input  ParamDataTypeStr=Inherit: Same as input
  to_kW : Gain  Gain=0.001
  State : Outport
  VehicleSpeed_[ms-1] : Outport  Port=2
  Vy_[ms-1] : Outport  Port=3
  ax_[ms-2] : Outport  Port=4
  ay_[ms-2] : Outport  Port=5
  PDrive_[kW] : Outport  Port=6
  TransmissionOut_[rpm] : Outport  Port=7
  wires:
  [vy] -> Vy_[ms-1]/1  "vy_[ms-1]"
  to_kW/1 -> PDrive_[kW]/1  "PDrive_[kW]"
  Gain/1 -> Product/1
  Bicycle_model_[XYZ]/10(ax_[ms-2]) -> ax_[ms-2]/1  "ax_[ms-2]"
  Product/1 -> to_kW/1
  [DT] -> Product/2
  Bicycle_model_[XYZ]/11(ay_[ms-2]) -> ay_[ms-2]/1  "ay_[ms-2]"
  Abs/1 -> Bicycle_model_[XYZ]/7(|vx|_[ms-1])
  Degrees to Radians/1 -> SteerRatio/1
  [vx] -> Abs/1
  SteerRatio/1 -> [DeltaWheel], Bicycle_model_[XYZ]/1(DeltaWheel_[rad])  "DeltaWheel_[rad]"
  TransmissionTorque_[Nm]/1 -> "FinalDriveRatio "/1  "DriveTorque_[Nm]"
  RearTyre/1(FyRear_[N]) -> Bicycle_model_[XYZ]/8(Fy_rear_[N])  "Fy_rear_[N]"
  FrontTyre/1(FyFront_[N]) -> Bicycle_model_[XYZ]/9(Fy_front_[N])  "Fy_front_[N]"
  Bicycle_model_[XYZ]/1(|vx|_[ms-1]1) -> [Absvx]  "|vx|_[ms-1]"
  Bicycle_model_[XYZ]/2(vy_[ms-1]) -> [vy], MuxDynState/2(vy [ms-1])  "Vy_[ms-1]"
  Bicycle_model_[XYZ]/4(RollAngle_[rad]) -> MuxDynState/4(R [rad]), [RollAngle]  "RollAngle_[rad]"
  Bicycle_model_[XYZ]/6(YawAngle_[rads-1]) -> [YawRate]  "YawRate_[rad s-1]"
  Bicycle_model_[XYZ]/7(Vx_[ms-1]) -> [vx]  "Vx_[ms-1]"
  [DeltaWheel] -> FrontTyre/1(DeltaWheel_[rad])
  [Absvx] -> FrontTyre/2(|vx|_[ms-1])
  [vy] -> FrontTyre/3(vy_[ms-1])
  [YawRate] -> FrontTyre/4(dYawAngle_[rads-1])
  [Absvx] -> RearTyre/1(|vx|_[ms-1])
  [vy] -> RearTyre/2(vy_[ms-1])
  [YawRate] -> RearTyre/3(dpsi_[rads-1])
  Bicycle_model_[XYZ]/3(vz_[ms-1]) -> MuxDynState/3(vz [ms-1])  "Vz_[ms-1]"
  Bicycle_model_[XYZ]/8(PitchAngle_[rad]) -> MuxDynState/5(P [rad])  "PitchAngle_[rad]"
  Bicycle_model_[XYZ]/9(YawAngle_[rad]) -> MuxDynState/6(Y [rad])  "YawAngle_[rad]"
  "[ms-1 --> rpm]"/1 -> Gain/1, FinalDriveRatio/1
  FinalDriveRatio/1 -> TransmissionOut_[rpm]/1  "TransmissionOut_[rpm]"
  [vx] -> "[ms-1 --> rpm]"/1, VehicleSpeed_[ms-1]/1, MuxDynState/1(vx [ms-1])  "vx_[ms-1]"
  [vx] -> Power Assisted Steering/1(Vx_[ms-1])
  DeltaSteer_[deg]/1 -> Power Assisted Steering/2(Delta_in_[deg])
  Power Assisted Steering/1(Delta_out_[deg]) -> Degrees to Radians/1
  [RollAngle] -> FrontTyre/5(RollAngle_[rad])
  [RollAngle] -> RearTyre/4(RollAngle_[rad])
  Constant3/1 -> Bicycle_model_[XYZ]/2(zFront_[m]_dzFront_[ms-1])  "zFront_[m]_dzFront_[m s-1]"
  Constant4/1 -> Bicycle_model_[XYZ]/3(zRear_[m]_dzRear_[ms-1])  "zRear_[m]_dzRear_[m s-1]"
  BrakePressure_[bar]/1 -> Bicycle_model_[XYZ]/4(BrakePressure_[bar])  "BrakePressure_[bar]"
  "FinalDriveRatio "/1 -> Bicycle_model_[XYZ]/5(DriveTorque_[Nm]), [DT]  "DriveTorque_[Nm]"
  Initial_Vx_[m s-1]/1 -> Bicycle_model_[XYZ]/6(v0_[ms-1])  "Initial_Vx_[m s-1]"
  Bicycle_model_[XYZ]/5(RollRate_[rads-1]) -> Terminator4/1  "RollRate_[rad s-1]"
  MuxDynState/1(State) -> State/1  "State"

== system EMPlanner_cs2018a/Audi_A8_Sedan_2/Dynamics_Simple/Engine ==
  ImpellerTorque_[Nm] : Inport
  Throttle_[%] : Inport  Port=2
  Configurable Subsystem : Subsystem  BlockChoice=Rate Limiter  mask{ComputationMode=ComputationMode}
      mask prompts: ComputationMode "Compuation mode:"
      mask init:
      | SetComputationMode(gcb,ComputationMode);
      settings: AttributesFormatString=%<BlockChoice>  OpenFcn=BringToFront(gcb);  MemberBlocks=Discrete Rate Limiter,Rate Limiter
      settings: TemplateBlock=|
      | PreScanSimulinkLibrary/Configurable Subsystems/TransferFunction
      | Engine/Configurable
      | Subsystem
  Configurable Subsystem1 : Subsystem  BlockChoice=Integrator  mask{ComputationMode=ComputationMode}
      mask prompts: ComputationMode "Computation mode:"
      mask init:
      | SetComputationMode(gcb,ComputationMode);
      settings: AttributesFormatString=%<BlockChoice>  OpenFcn=BringToFront(gcb);  MemberBlocks=Discrete-Time Integrator,Integrator
      settings: TemplateBlock=|
      | PreScanSimulinkLibrary/Configurable Subsystems/integral with initial condition and limts
      | for engine/Configurable
      | Subsystem
  EngineTorque : Lookup2D  RowIndex=p.thvec  ColumnIndex=p.nevec  Table=p.emap  InputSameDT=on
  Gain : Gain  Gain=2*pi/60
  Product : Product  RndMeth=Zero
  Sum : Sum  Inputs=-+  InputSameDT=on  SaturateOnIntegerOverflow=on  OutDataTypeStr=Inherit: Same as first input
  engine + impeller inertia : Gain  Gain=1/p.Iei  SaturateOnIntegerOverflow=on  OutDataTypeStr=Inherit: Same as input  ParamDataTypeStr=Inherit: Same as input
  rad|sec2rpm : Gain  Gain=60/2/pi  SaturateOnIntegerOverflow=on  OutDataTypeStr=Inherit: Same as input  ParamDataTypeStr=Inherit: Same as input
  to_kW : Gain  Gain=0.001
  nEngine_[rpm] : Outport  InitialOutput=0
  PEngine_[kW] : Outport  Port=2  InitialOutput=0
  wires:
  rad|sec2rpm/1 -> nEngine_[rpm]/1, EngineTorque/2, Gain/1  "rpm"
  engine + impeller inertia/1 -> Configurable Subsystem1/1(In1)  "rads-2"
  EngineTorque/1 -> Sum/2, Product/2
  Sum/1 -> engine + impeller inertia/1
  Configurable Subsystem1/1(Out1) -> rad|sec2rpm/1  "rads-1"
  Throttle_[%]/1 -> Configurable Subsystem/1(In1)
  ImpellerTorque_[Nm]/1 -> Sum/1
  Configurable Subsystem/1(Out1) -> EngineTorque/1
  Product/1 -> to_kW/1
  Gain/1 -> Product/1
  to_kW/1 -> PEngine_[kW]/1

== system EMPlanner_cs2018a/Audi_A8_Sedan_2/Dynamics_Simple/Gear: Auto Manual ==
  note: 0; Auto = on // Manual =off
      | 1; Auto = off // Manual =on
  Auto_Manual : Inport
  Manual_Gear : Inport  Port=2
  Auto_Gear : Inport  Port=3
  If : If  IfExpression=u1 == 0
  If Action Subsystem : Subsystem  TreatAsAtomicUnit=on
  If Action Subsystem1 : Subsystem  TreatAsAtomicUnit=on
  Merge : Merge
  Gear : Outport
  wires:
  If Action Subsystem/1(Out1) -> Merge/1
  Auto_Gear/1 -> If Action Subsystem/1(In1)
  If/1 -> If Action Subsystem/Action
  Merge/1 -> Gear/1
  If Action Subsystem1/1(Out1) -> Merge/2
  Manual_Gear/1 -> If Action Subsystem1/1(In1)
  If/2 -> If Action Subsystem1/Action
  Auto_Manual/1 -> If/1

== system EMPlanner_cs2018a/Audi_A8_Sedan_2/Dynamics_Simple/ShiftLogic ==
  Throttle_[%] : Inport
  GearNr_[-] : Inport  Port=2
  Auto_GearShift : Inport  Port=3
  VehSpeed_[ms-1] : Inport  Port=4
  Add2 : Sum
  Data Type Conversion1 : DataTypeConversion  OutDataTypeStr=double
  Detect Increase1 : simulink/Logic and Bit Operations/Detect Increase  vinit=0.0  OutDataTypeStr=uint8
  Detect Increase : Subsystem
  Gear limitation : Saturate  UpperLimit=p.maxGear  LowerLimit=1
  Gear limitation while shifting : Saturate  UpperLimit=p.maxGear  LowerLimit=1
  GearNeutral : Constant  Value=0
  GearReverse : Constant  Value=-1
  "IC, gear = 1" : Memory  InitialCondition=1  InheritSampleTime=on
  If Action Neutral : Subsystem  TreatAsAtomicUnit=on
  If Action Normal : Subsystem  TreatAsAtomicUnit=on
  If Action Reverse : Subsystem  TreatAsAtomicUnit=on
  Memory : Memory  InheritSampleTime=on
  Merge : Merge  Inputs=3
  Relational Operator : RelationalOperator  OutDataTypeStr=boolean  RndMeth=Nearest
  Relational Operator1 : RelationalOperator  Operator=<=  OutDataTypeStr=boolean  RndMeth=Nearest
  Shift_Down time : Delay  DelayLength=p.ShiftDown_fac
  Shift_Up time : Delay  DelayLength=p.ShiftUp_fac
  Sum : Sum  Inputs=+-
  interp_down : Lookup2D  RowIndex=p.downth  ColumnIndex=[1:p.maxGear]  Table=p.downtab  LookUpMeth=Interpolation-Use End Values  InputSameDT=on
  interp_up : Lookup2D  RowIndex=p.upth  ColumnIndex=[1:p.maxGear]  Table=p.uptab  LookUpMeth=Interpolation-Use End Values  InputSameDT=on
  reverse/neutral/normal gear : If  IfExpression=u1 == 0  ElseIfExpressions=u1 < 0
  to_ms-1 : Gain  Gain=1/3.6
  "to_ms-1 " : Gain  Gain=1/3.6
  GearNr : Outport
  wires:
  Auto_GearShift/1 -> reverse/neutral/normal gear/1
  "IC, gear = 1"/1 -> If Action Normal/1(In1)
  Merge/1 -> GearNr/1
  If Action Reverse/1(Out1) -> Merge/2
  If Action Neutral/1(Out1) -> Merge/1
  If Action Normal/1(Out1) -> Merge/3
  reverse/neutral/normal gear/3 -> If Action Normal/Action
  reverse/neutral/normal gear/1 -> If Action Neutral/Action
  reverse/neutral/normal gear/2 -> If Action Reverse/Action
  GearReverse/1 -> If Action Reverse/1(In1)
  GearNeutral/1 -> If Action Neutral/1(In1)
  Shift_Down time/1 -> Sum/2
  Shift_Up time/1 -> Sum/1
  Detect Increase/1(Out1) -> Shift_Up time/1
  Data Type Conversion1/1 -> Shift_Down time/1
  Detect Increase1/1 -> Data Type Conversion1/1
  Sum/1 -> Add2/1
  Memory/1 -> Add2/2  "GearNr_[-]"
  Add2/1 -> Gear limitation while shifting/1
  Gear limitation while shifting/1 -> "IC, gear = 1"/1, Memory/1  "GearNr_[-]"
  Throttle_[%]/1 -> interp_down/1, interp_up/1
  Relational Operator/1 -> Detect Increase/2(In2)
  Relational Operator1/1 -> Detect Increase1/1
  interp_down/1 -> "to_ms-1 "/1
  VehSpeed_[ms-1]/1 -> Relational Operator/1, Relational Operator1/1
  interp_up/1 -> to_ms-1/1
  Gear limitation/1 -> interp_down/2, interp_up/2, Detect Increase/1(GearNr_[-])
  GearNr_[-]/1 -> Gear limitation/1
  to_ms-1/1 -> Relational Operator/2
  "to_ms-1 "/1 -> Relational Operator1/2

== system EMPlanner_cs2018a/Audi_A8_Sedan_2/Dynamics_Simple/Transmission ==
  nEngine_[rpm] : Inport
  GearNr_[-] : Inport  Port=2
  n_TransmissionOut_[rpm] : Inport  Port=3
  Torque_Converter : Subsystem
      mask Display: image(imread('TorqueConverter.png'));
  Transmission_Ratio : Subsystem
  Viscous coupling : Lookup  InputValues=[-5:0.1:5]*p.m/4  Table=p.m/4*tanh([-5:0.1:5])
  ImpellerTorque_[Nm] : Outport  InitialOutput=0
  TransmissionTorque_[Nm] : Outport  Port=2  InitialOutput=0
  wires:
  Torque_Converter/2(TurbineTorque_[Nm]) -> Viscous coupling/1  "Converter_Torque_[Nm]"
  Transmission_Ratio/2(nTransmissionIn_[rpm]) -> Torque_Converter/2(nTransmission_[rpm])
  nEngine_[rpm]/1 -> Torque_Converter/1(nEngine_[rpm])
  GearNr_[-]/1 -> Transmission_Ratio/2(GearNr_[-]), Torque_Converter/3(Gear nr)
  n_TransmissionOut_[rpm]/1 -> Transmission_Ratio/3(nTransmissionOut_[rpm])
  Torque_Converter/1(ImpellerTorque_[Nm]) -> ImpellerTorque_[Nm]/1
  Transmission_Ratio/1(tTransmissionOut_[Nm]) -> TransmissionTorque_[Nm]/1
  Viscous coupling/1 -> Transmission_Ratio/1(tTransmissionIn_[Nm])
